simulink model "PD_G"  (R2021a)
settings: Solver=VariableStepAuto  StartTime=0.0  StopTime=100.0  RelTol=1e-3
values from neighbouring files (symbols this model uses):
  kd = eye(3)*4    [params.m]
  kp = eye(3)*50    [params.m]
settings Model: Creator=antoninoparisi  LastModifiedBy=antoninoparisi

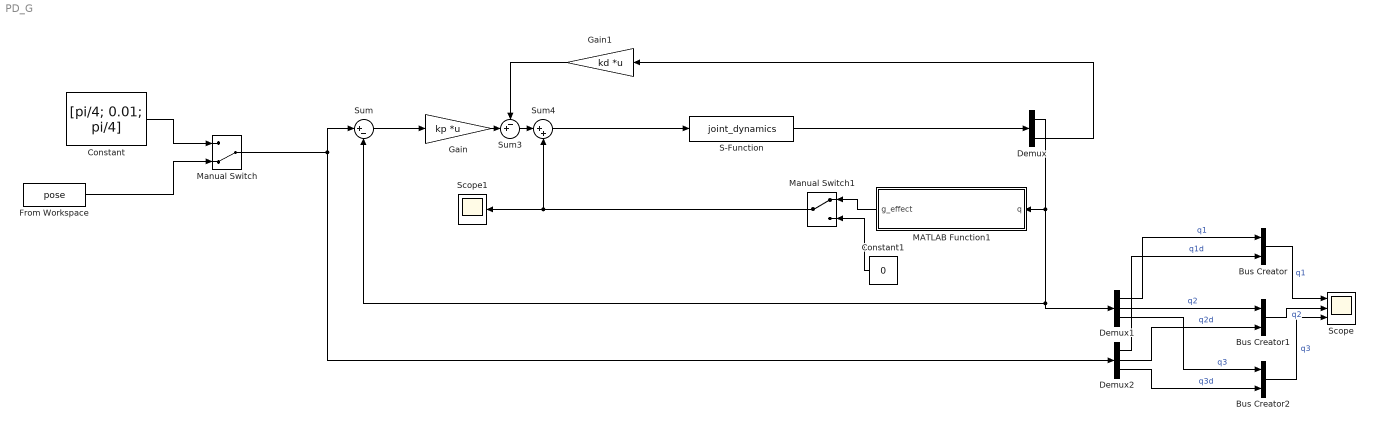
== system PD_G ==
  Bus Creator : BusCreator  Inputs=2
  Bus Creator1 : BusCreator  Inputs=2
  Bus Creator2 : BusCreator  Inputs=2
  Constant : Constant  Value=[pi/4; 0.01; pi/4]  VectorParams1D=off
  Constant1 : Constant  Value=0
  Demux : Demux  Outputs=2
  Demux1 : Demux  Outputs=3
  Demux2 : Demux  Outputs=3
  From Workspace : FromWorkspace  VariableName=pose
  Gain : Gain  Gain=kp  Multiplication=Matrix(K*u) (u vector)
  Gain1 : Gain  Gain=kd  Multiplication=Matrix(K*u) (u vector)
  MATLAB Function1 : MATLAB Function  TreatAsAtomicUnit=on
  Manual Switch : ManualSwitch  CurrentSetting=0
  Manual Switch1 : ManualSwitch
  S-Function : S-Function  FunctionName=joint_dynamics  Parameters=robot  SFunctionDeploymentMode=off  EnableBusSupport=off
  Scope : Scope  NumInputPorts=3
  Scope1 : Scope
  Sum : Sum  Inputs=|+-
  Sum3 : Sum  Inputs=-+|
  Sum4 : Sum  Inputs=|++
  wires:
  Manual Switch/1 -> Sum/1, Demux2/1
  S-Function/1 -> Demux/1
  Gain/1 -> Sum3/2
  Gain1/1 -> Sum3/1
  Sum3/1 -> Sum4/1
  Sum4/1 -> S-Function/1
  Demux/2 -> Gain1/1
  Sum/1 -> Gain/1
  Demux/1 -> MATLAB Function1/1(q), Demux1/1, Sum/2
  Bus Creator1/1 -> Scope/2  "q2"
  Bus Creator2/1 -> Scope/3  "q3"
  Bus Creator/1 -> Scope/1  "q1"
  Demux1/1 -> Bus Creator/1  "q1"
  Demux2/1 -> Bus Creator/2  "q1d"
  Demux1/2 -> Bus Creator1/1  "q2"
  Demux2/2 -> Bus Creator1/2  "q2d"
  Demux2/3 -> Bus Creator2/2  "q3d"
  Demux1/3 -> Bus Creator2/1  "q3"
  Constant/1 -> Manual Switch/1
  From Workspace/1 -> Manual Switch/2
  MATLAB Function1/1(g_effect) -> Manual Switch1/1
  Constant1/1 -> Manual Switch1/2
  Manual Switch1/1 -> Sum4/2, Scope1/1

== matlab function PD_G/MATLAB Function1 ==
  data: q input size=3; g_effect output size=3
function g_effect = gravity(q)

g_effect = G_Lagrangian(q);
